simulink model "Driving_dynamics_model"  (R2025a)
settings: Solver=VariableStepAuto  StartTime=0.0  StopTime=20  RelTol=1e-3
values from neighbouring files (symbols this model uses):
  a = 1.8    [Longitdunal_driving_parameters.m]    (also in Longitudinal_driving_parametrs.m)
  A = 1.25    [Longitdunal_driving_parameters.m]    (also in Longitudinal_driving_parametrs.m)
  a1 = -1e-5    (= -1e-05)    [Longitdunal_driving_parameters.m]    (also in Longitudinal_driving_parametrs.m)
  a2 = 1.25    [Longitdunal_driving_parameters.m]    (also in Longitudinal_driving_parametrs.m)
  B = 5.7507    [Longitdunal_driving_parameters.m]    (also in Longitudinal_driving_parametrs.m = 4.1576)
  C = 1.2421    [Longitdunal_driving_parameters.m]    (also in Longitudinal_driving_parametrs.m = 1.718)
  cd = 0.4    [Longitdunal_driving_parameters.m]    (also in Longitudinal_driving_parametrs.m)
  cz = 1    [Longitdunal_driving_parameters.m]    (also in Longitudinal_driving_parametrs.m)
  enginemap = [-0.15, 0.23, 0.60, 0.68, 0.8 ... (first row only)    [Longitdunal_driving_parameters.m]
  enginerpm = linspace(1000,15000,15)'    [Longitdunal_driving_parameters.m]
  g = 9.81    [Longitdunal_driving_parameters.m]    (also in Longitudinal_driving_parametrs.m)
  h = 0.2    [Longitdunal_driving_parameters.m]    (also in Longitudinal_driving_parametrs.m)
  igear = [23.10,17.64, 13.86, 10.92, 8.82, 7.14, 5.88, 4.33]'    [Longitdunal_driving_parameters.m]    (also in Longitudinal_driving_parametrs.m = [23.10,17.64,13.86])
  Iwheel = 0.9    [Longitdunal_driving_parameters.m]
  L = 3.5    [Longitdunal_driving_parameters.m]    (also in Longitudinal_driving_parametrs.m)
  m = 850    [Longitdunal_driving_parameters.m]    (also in Longitudinal_driving_parametrs.m)
  r = 0.375    [Longitdunal_driving_parameters.m]    (also in Longitudinal_driving_parametrs.m)
  rho = 1.225    [Longitdunal_driving_parameters.m]    (also in Longitudinal_driving_parametrs.m)
  rpm_idling = 1000    [Longitdunal_driving_parameters.m]
  rpm_limit = 15000    [Longitdunal_driving_parameters.m]
  rpm_up = 13500    [Longitdunal_driving_parameters.m]
  TengMax = 250    [Longitdunal_driving_parameters.m]
  throttlepos = [0, 0.25, 0.5, 0.75, 1]'    [Longitdunal_driving_parameters.m]
settings Model: Creator=g.m.morjaria  LastModifiedBy=g.m.morjaria

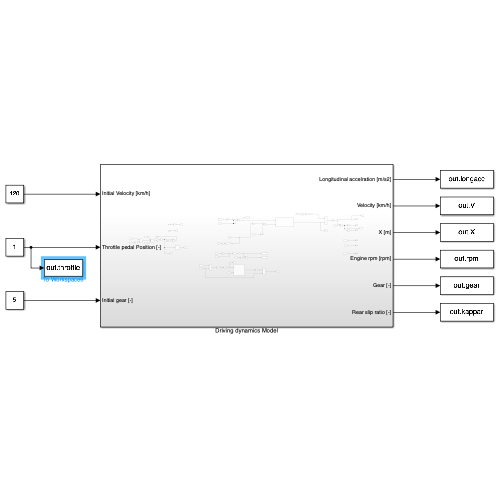
[thumbnail: Simulink's stored preview of the top-level diagram]
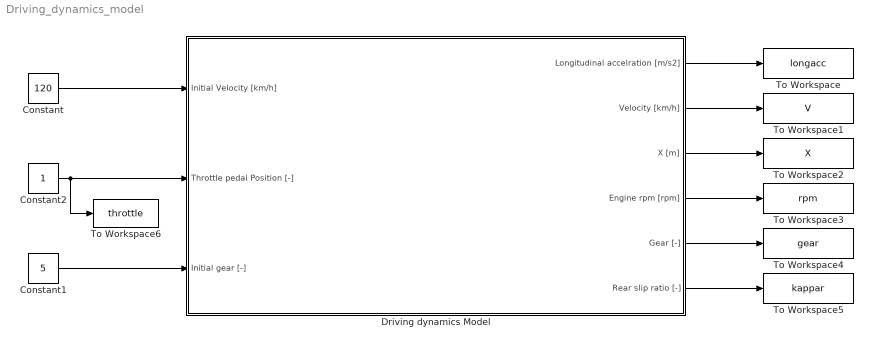
== system Driving_dynamics_model ==
  Constant : Constant  Value=120
  Constant1 : Constant  Value=5
  Constant2 : Constant
  Driving dynamics Model : Subsystem
  To Workspace : ToWorkspace  VariableName=longacc  SaveFormat=Timeseries  SampleTime=-1
  To Workspace1 : ToWorkspace  VariableName=V  SaveFormat=Timeseries  SampleTime=-1
  To Workspace2 : ToWorkspace  VariableName=X  SaveFormat=Timeseries  SampleTime=-1
  To Workspace3 : ToWorkspace  VariableName=rpm  SaveFormat=Timeseries  SampleTime=-1
  To Workspace4 : ToWorkspace  VariableName=gear  SaveFormat=Timeseries  SampleTime=-1
  To Workspace5 : ToWorkspace  VariableName=kappar  SaveFormat=Timeseries  SampleTime=-1
  To Workspace6 : ToWorkspace  VariableName=throttle  SaveFormat=Timeseries  SampleTime=-1
  wires:
  Driving dynamics Model/1(Longitudinal accelration [m/s2]) -> To Workspace/1
  Driving dynamics Model/6(Rear slip ratio [-]) -> To Workspace5/1
  Driving dynamics Model/5(Gear [-]) -> To Workspace4/1
  Driving dynamics Model/4(Engine rpm [rpm]) -> To Workspace3/1
  Driving dynamics Model/3(X [m]) -> To Workspace2/1
  Driving dynamics Model/2(Velocity [km/h]) -> To Workspace1/1
  Constant/1 -> Driving dynamics Model/1(Initial Velocity [km/h])
  Constant1/1 -> Driving dynamics Model/3(Initial gear [-])
  Constant2/1 -> To Workspace6/1, Driving dynamics Model/2(Throttle pedal Position [-])

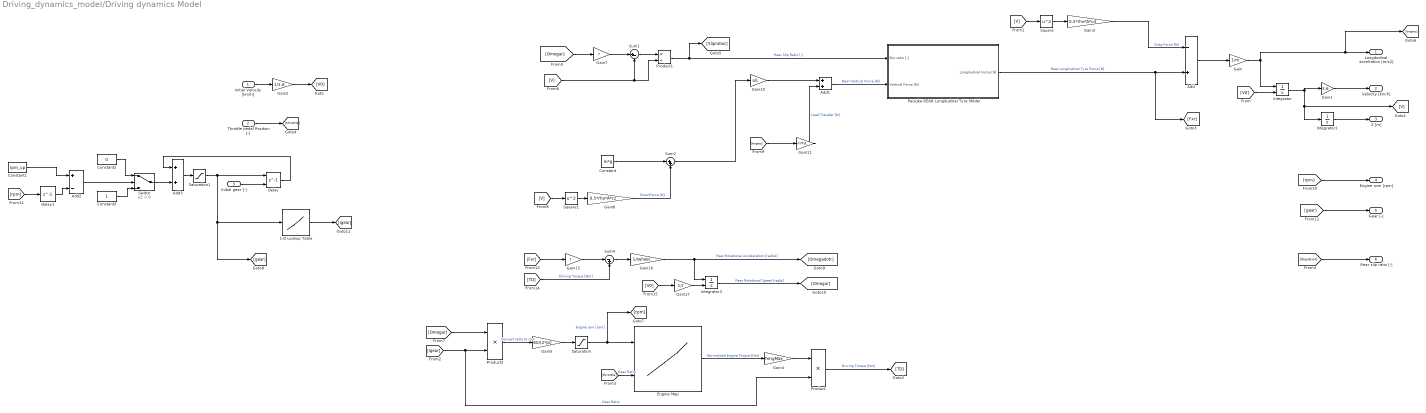
== system Driving_dynamics_model/Driving dynamics Model ==
  Initial Velocity [km/h] : Inport
  Throttle pedal Position [-] : Inport  Port=2
  Initial gear [-] : Inport  Port=3
  1-D Lookup Table : Lookup_n-D  NumberOfTableDimensions=1  BreakpointsForDimension1=[1:8]  Table=igear  InternalRulePriority=Speed  RndMeth=Simplest
  Add : Sum  Inputs=-+
  Add1 : Sum
  Add2 : Sum  Inputs=+-
  Add3 : Sum
  Constant : Constant  Value=m*g
  Constant1 : Constant  Value=rpm_up
  Constant2 : Constant  Value=0
  Constant3 : Constant
  Delay : Delay  DelayLength=1  InitialConditionSource=Input port  InputProcessing=Columns as channels (frame based)
      settings: InputPortMap=u0,p4
  Delay1 : Delay  DelayLength=1  InputProcessing=Columns as channels (frame based)
  Engine Map : Lookup_n-D  BreakpointsForDimension1=enginerpm  BreakpointsForDimension2=throttlepos  Table=enginemap  InternalRulePriority=Speed  RndMeth=Simplest
      settings: InputPortMap=u0,u1
  Gain : Gain  Gain=1/m
  Gain1 : Gain  Gain=3.6
  Gain10 : Gain  Gain=a/L
  Gain11 : Gain  Gain=m*h/L
  Gain15 : Gain  Gain=r
  Gain16 : Gain  Gain=1/Iwheel
  Gain17 : Gain  Gain=1/r
  Gain2 : Gain  Gain=1/3.6
  Gain3 : Gain  Gain=0.5*rho*A*cd
  Gain4 : Gain  Gain=TengMax
  Gain5 : Gain  Gain=60/(2*pi)
  Gain7 : Gain  Gain=r
  Gain8 : Gain  Gain=0.5*rho*A*cz
  Integrator : Integrator  InitialConditionSource=external
  Integrator1 : Integrator
  Integrator3 : Integrator  InitialConditionSource=external
  Pacejka REAR Longitudinal Tyre Model : Subsystem
  Product : Product  Inputs=**
  Product1 : Product  Inputs=*/
  Product2 : Product  Inputs=**
  Saturation : Saturate  UpperLimit=rpm_limit  LowerLimit=rpm_idling
  Saturation1 : Saturate  UpperLimit=length(igear)  LowerLimit=1
  Square : Math  Operator=square
  Square1 : Math  Operator=square
  Sum1 : Sum  Inputs=|+-
  Sum2 : Sum  Inputs=|++
  Sum4 : Sum  Inputs=|-+
  Switch : Switch  Criteria=u2 > Threshold  SaturateOnIntegerOverflow=off  InputSameDT=off
  Longitudinal accelration [m/s2] : Outport
  Velocity [km/h] : Outport  Port=2
  X [m] : Outport  Port=3
  Engine rpm [rpm] : Outport  Port=4
  Gear [-] : Outport  Port=5
  Rear slip ratio [-] : Outport  Port=6
  wires:
  Square/1 -> Gain3/1
  Add1/1 -> Pacejka REAR Longitudinal Tyre Model/2(Vertical Force [N])  "Rear Vertical Force [N]"
  [Fxr] -> Gain15/1
  Gain16/1 -> [Omegadotr], Integrator3/1  "Rear Rotational Acceleration [rad/s2]"
  Gain15/1 -> Sum4/1
  [V0] -> Gain17/1
  [Omegar] -> Gain7/1
  Gain8/1 -> Sum2/2  "DownForce [N]"
  Add/1 -> Gain/1
  Square1/1 -> Gain8/1
  Gain17/1 -> Integrator3/2
  Gain3/1 -> Add/1  "Drag Force [N]"
  [TD] -> Sum4/2  "Driving Torque [Nm]"
  Sum2/1 -> Gain10/1
  Gain11/1 -> Add1/2  "Load Transfer [N]"
  Gain2/1 -> [V0]
  [V0] -> Integrator/2
  Integrator3/1 -> [Omegar]  "Rear Rotational Speed [rad/s]"
  Initial Velocity [km/h]/1 -> Gain2/1
  Gain1/1 -> Velocity [km/h]/1
  Sum1/1 -> Product1/1
  Sum4/1 -> Gain16/1
  Gain/1 -> [longacc], Longitudinal accelration [m/s2]/1, Integrator/1
  Constant/1 -> Sum2/1
  [V] -> Square1/1
  Integrator1/1 -> X [m]/1
  Integrator/1 -> Gain1/1, [V], Integrator1/1
  Product1/1 -> Pacejka REAR Longitudinal Tyre Model/1(Slip ratio [-]), [Slipratior]  "Rear Slip Ratio [-]"
  Pacejka REAR Longitudinal Tyre Model/1(Longitudinal Force [N]) -> [Fxr], Add/2  "Rear Longitudinal Tyre Force [N]"
  [longacc] -> Gain11/1
  [V] -> Square/1
  Gain10/1 -> Add1/1
  [V] -> Product1/2, Sum1/2
  Gain7/1 -> Sum1/1
  [Slipratior] -> Rear slip ratio [-]/1
  Engine Map/1 -> Gain4/1  "Normalised Engine Torque [Nm]"
  Gain4/1 -> Product/1
  [igear] -> Product2/2, Product/2  "Gear Ratio"
  Product/1 -> [TD]  "Driving Torque [Nm]"
  [throttle] -> Engine Map/2  "Gear Ratio"
  Throttle pedal Position [-]/1 -> [throttle]
  [Omegar] -> Product2/1
  Product2/1 -> Gain5/1  "Convert rad/s to rpm"
  [rpm] -> Engine rpm [rpm]/1
  Gain5/1 -> Saturation/1
  Saturation/1 -> [rpm], Engine Map/1  "Engine rpm [rpm]"
  Constant1/1 -> Add2/1
  Add2/1 -> Switch/2
  Constant2/1 -> Switch/1
  Constant3/1 -> Switch/3
  Switch/1 -> Add3/2
  Add3/1 -> Saturation1/1
  Delay/1 -> Add3/1
  Initial gear [-]/1 -> Delay/2
  Delay1/1 -> Add2/2
  [rpm] -> Delay1/1
  1-D Lookup Table/1 -> [igear]
  Saturation1/1 -> 1-D Lookup Table/1, [gear], Delay/1
  [gear] -> Gear [-]/1

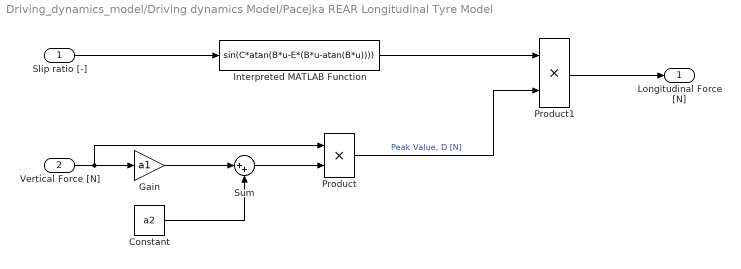
== system Driving_dynamics_model/Driving dynamics Model/Pacejka REAR Longitudinal Tyre Model ==
  Slip ratio [-] : Inport
  Vertical Force [N] : Inport  Port=2
  Constant : Constant  Value=a2
  Gain : Gain  Gain=a1
  Interpreted MATLAB Function : MATLABFcn  MATLABFcn=sin(C*atan(B*u-E*(B*u-atan(B*u))))
  Product : Product
  Product1 : Product
  Sum : Sum  Inputs=|++
  Longitudinal Force [N] : Outport
  wires:
  Product1/1 -> Longitudinal Force [N]/1
  Interpreted MATLAB Function/1 -> Product1/1
  Slip ratio [-]/1 -> Interpreted MATLAB Function/1
  Product/1 -> Product1/2  "Peak Value, D [N]"
  Sum/1 -> Product/2
  Constant/1 -> Sum/2
  Gain/1 -> Sum/1
  Vertical Force [N]/1 -> Gain/1, Product/1
